simulink model "Quanser_Qube_Plant_LQR_Upright"  (R2019a)
settings: Solver=VariableStepAuto  StartTime=0.0  StopTime=10.0  RelTol=1e-3
values from neighbouring files (symbols this model uses):
  Klqr = [35, -2, 3, -1.5 ]    [parametric_systemID_upright.m]    (also in uprightController.m = Klqr')
libraries: cstblocks x3, simulink x1
settings Model: Creator=emma  LastModifiedBy=emma

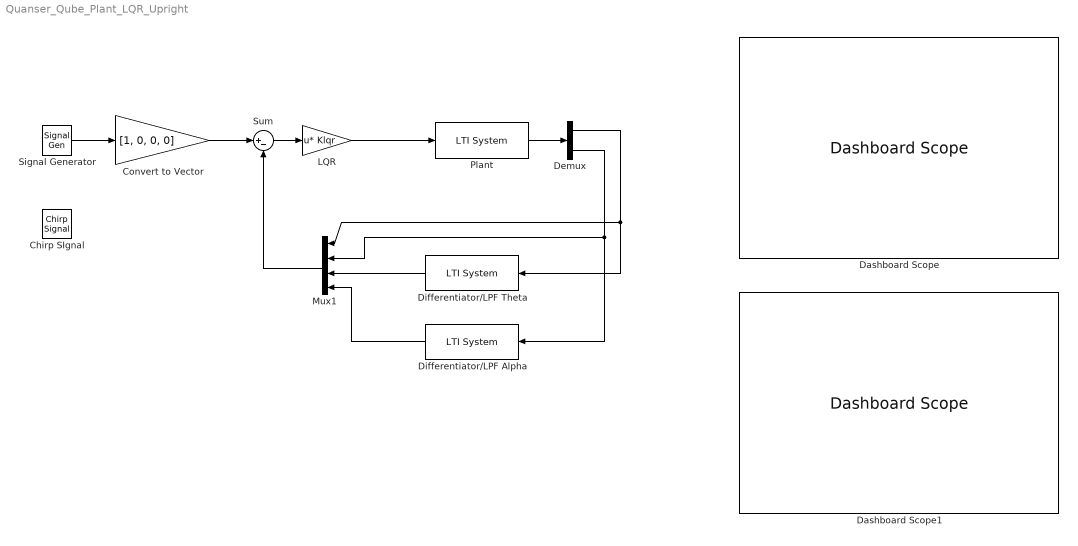
== system Quanser_Qube_Plant_LQR_Upright ==
  Chirp SIgnal : simulink/Sources/Chirp Signal  f1=0.1  T=10  f2=100
  Convert to Vector : Gain  Gain=[1, 0, 0, 0]
  Dashboard Scope : DashboardScope
  Dashboard Scope1 : DashboardScope
  Demux : Demux  Outputs=2
  Differentiator/LPF Alpha : cstblocks/LTI System  sys=Diff_LPF  IC=[]
  Differentiator/LPF Theta : cstblocks/LTI System  sys=Diff_LPF  IC=[]
  LQR : Gain  Gain=Klqr  Multiplication=Matrix(u*K)
  Mux1 : Mux
  Plant : cstblocks/LTI System  sys=Galt  IC=[]
  "Signal Generator " : SignalGenerator  Frequency=6.28  Units=rad/sec  VectorParams1D=off
  Sum : Sum  Inputs=|+-
  wires:
  "Signal Generator "/1 -> Convert to Vector/1
  Plant/1 -> Demux/1
  Demux/1 -> Differentiator/LPF Theta/1, Mux1/1
  Demux/2 -> Differentiator/LPF Alpha/1, Mux1/2
  LQR/1 -> Plant/1
  Sum/1 -> LQR/1
  Convert to Vector/1 -> Sum/1
  Differentiator/LPF Theta/1 -> Mux1/3
  Mux1/1 -> Sum/2
  Differentiator/LPF Alpha/1 -> Mux1/4
